simulink model "SEA_control_loop"  (R2015a)
settings: Solver=ode45  StartTime=0.0  StopTime=10.0  RelTol=1e-3
undefined symbols (not defined in the file or in its folder): fdesignblkfcn, gcbh, k_spring, sample_time
settings Model: Creator=wmartin  LastModifiedBy=wmartin

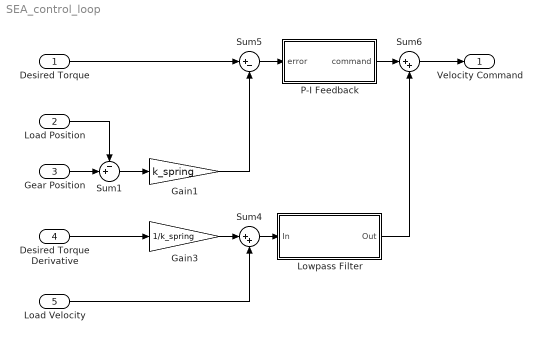
== system SEA_control_loop ==
  Desired Torque : Inport
  Load Position : Inport  Port=2
  Gear Position : Inport  Port=3
  Desired Torque Derivative : Inport  Port=4
  Load Velocity : Inport  Port=5
  Gain1 : Gain  Gain=k_spring
  Gain3 : Gain  Gain=1/k_spring
  Lowpass Filter : Subsystem  DialogController=fdesignblkfcn  InitFcn=fdesignblkfcn(gcbh, {'InitFcn'});  mask(Lowpass Filter){}
      mask help: Design a lowpass filter
      settings: CopyFcn=fdesignblkfcn(gcbh, {'CopyFcn'});
      mask Help: helpview(mapfilelocation('dsp'), 'dsplowpassfilter');
      mask Display: disp('Lowpass')
  P-I Feedback : Subsystem
  Sum1 : Sum  Inputs=-+|
  Sum4 : Sum  Inputs=|++
  Sum5 : Sum  Inputs=|+-
  Sum6 : Sum  Inputs=|++
  Velocity Command : Outport
  wires:
  Gain1/1 -> Sum5/2
  Load Position/1 -> Sum1/1
  Gear Position/1 -> Sum1/2
  Desired Torque/1 -> Sum5/1
  Sum6/1 -> Velocity Command/1
  Gain3/1 -> Sum4/1
  Desired Torque Derivative/1 -> Gain3/1
  Load Velocity/1 -> Sum4/2
  Sum4/1 -> Lowpass Filter/1(In)
  Lowpass Filter/1(Out) -> Sum6/2
  Sum1/1 -> Gain1/1
  Sum5/1 -> P-I Feedback/1(error)
  P-I Feedback/1(command) -> Sum6/1

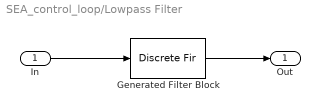
== system SEA_control_loop/Lowpass Filter ==
  In : Inport
  Generated Filter Block : DiscreteFir  Tag=BlockMethodSubSystem  Coefficients=[-0.049792265798371309 -0.00478204397482343 -0.0023545966524627579 0.0019617877955006649 0.0081617445920188422 0.01606136498204886 0.025426522925330174 0.035808512742994333 0.046780148761454213 0.057713212050140641 0.068077289761393753 0.077169075575072327 0.084565882051693325 0.089692876147162801 0.092473878579640248 0.092473878579640248 0.089692876147162801 0.084565882051693325 0.077169075575072327 0.068077289761393753 0.057713212050140641 0.046780148761454213 0.035808512742994333 0.025426522925330174 0.01606136498204886 0.0081617445920188422 0.0019617877955006649 -0.0023545966524627579 -0.00478204397482343 -0.049792265798371309]
  Out : Outport
  wires:
  In/1 -> Generated Filter Block/1
  Generated Filter Block/1 -> Out/1

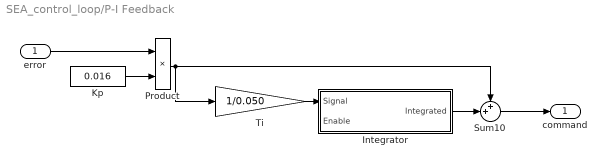
== system SEA_control_loop/P-I Feedback ==
  error : Inport
  Integrator : Subsystem
  Kp : Constant  Value=0.016
  Product : Product
  Sum10 : Sum  Inputs=++|
  Ti : Gain  Gain=1/0.050
  command : Outport
  wires:
  ? -> Integrator/2(Enable)
  Sum10/1 -> command/1
  Product/1 -> Ti/1, Sum10/1
  Kp/1 -> Product/2
  error/1 -> Product/1
  Integrator/1(Integrated) -> Sum10/2
  Ti/1 -> Integrator/1(Signal)

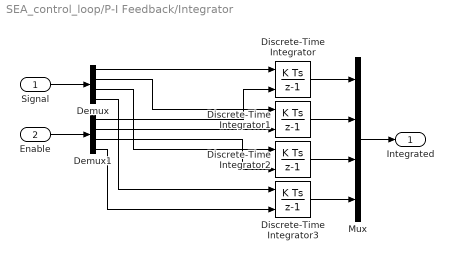
== system SEA_control_loop/P-I Feedback/Integrator ==
  Signal : Inport
  Enable : Inport  Port=2
  Demux : Demux
  Demux1 : Demux
  Discrete-Time Integrator{,1..3} (4 alike) : DiscreteIntegrator  ExternalReset=rising  InitialConditionSetting=State (most efficient)  SampleTime=sample_time  LimitOutput=on  UpperSaturationLimit=1  LowerSaturationLimit=-1
  Mux : Mux
  Integrated : Outport
  wires:
  Signal/1 -> Demux/1
  Discrete-Time Integrator/1 -> Mux/1
  Enable/1 -> Demux1/1
  Mux/1 -> Integrated/1
  Discrete-Time Integrator1/1 -> Mux/2
  Discrete-Time Integrator2/1 -> Mux/3
  Discrete-Time Integrator3/1 -> Mux/4
  Demux1/4 -> Discrete-Time Integrator3/2
  Demux1/3 -> Discrete-Time Integrator2/2
  Demux1/2 -> Discrete-Time Integrator1/2
  Demux1/1 -> Discrete-Time Integrator/2
  Demux/1 -> Discrete-Time Integrator/1
  Demux/2 -> Discrete-Time Integrator1/1
  Demux/3 -> Discrete-Time Integrator2/1
  Demux/4 -> Discrete-Time Integrator3/1
